simulink model "SystemIDsimulink"  (R2024b)
settings: Solver=ode5  StartTime=0.0  StopTime=20  FixedStep=.0005  RelTol=1e-3
undefined symbols (not defined in the file or in its folder): National_Instruments, PCIe
libraries: sldrtlib x4, slident x1, simulink x1
settings Model: Creator=jcglenn  LastModifiedBy=jcglenn
settings HardwareCC: ProdBitPerLong=64  ProdHWDeviceType=Intel->x86-64 (Linux 64)
settings RTWCC: Description=Simulink Desktop Real-Time  SystemTargetFile=sldrt.tlc  TemplateMakefile=sldrt.tmf  RTWCompilerOptimization=on
settings CodeAppCC: MaxIdLength=95
settings SimulinkDesktopRealTimeCC: TargetLibSuffix=_sldrt.a  TargetPreCompLibLocation=C:\Program Files\MATLAB\R2024b\toolbox\sldrt\lib\win64  ParMdlRefBuildCompliant=on

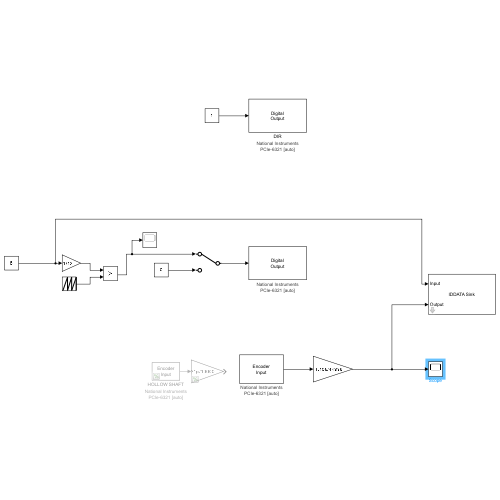
[thumbnail: Simulink's stored preview of the top-level diagram]
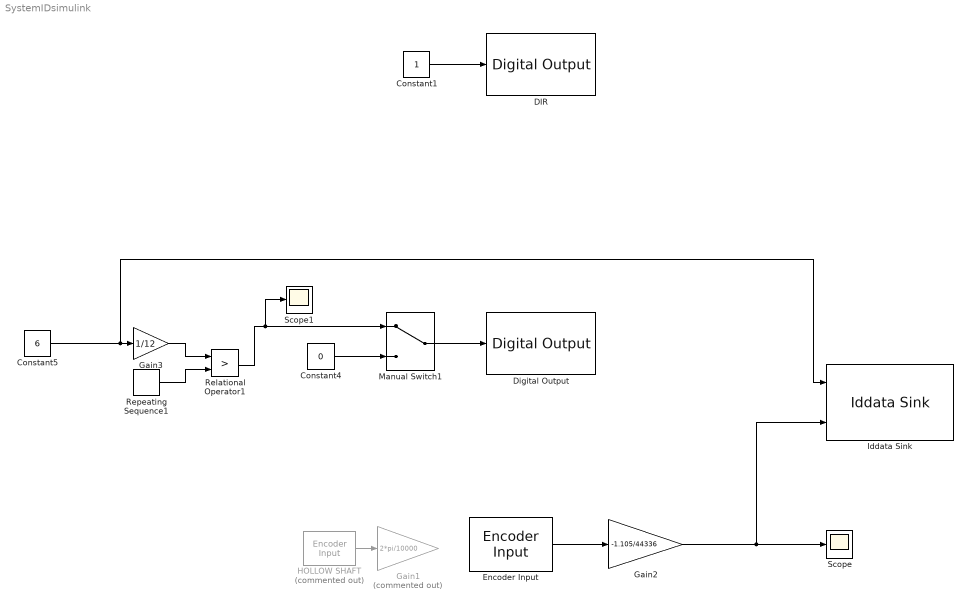
== system SystemIDsimulink ==
  Constant1 : Constant
  Constant4 : Constant  Value=0
  Constant5 : Constant  Value=6
  DIR : sldrtlib/Digital Output  SampleTime=0.0005  MaxMissedTicks=1000  ShowMissedTicks=off  YieldWhenWaiting=off  DrvName=National_Instruments/PCIe-6321  DrvAddress=4294967295  DrvOptions=[0 3 0 2 2 0 0]  Channels=2  BitMode=1  InitialValue=[]  FinalValue=[]
      settings: AttributesFormatString=National Instruments\nPCIe-6321 [auto]
  Digital Output : sldrtlib/Digital Output  SampleTime=0.0005  MaxMissedTicks=1000  ShowMissedTicks=off  YieldWhenWaiting=off  DrvName=National_Instruments/PCIe-6321  DrvAddress=4294967295  DrvOptions=[0 3 0 2 2 0 0]  Channels=1  BitMode=1  InitialValue=[]  FinalValue=[]
      settings: AttributesFormatString=National Instruments\nPCIe-6321 [auto]
  Encoder Input : sldrtlib/Encoder Input  SampleTime=0.0005  MaxMissedTicks=1000  ShowMissedTicks=off  YieldWhenWaiting=off  DrvName=National_Instruments/PCIe-6321  DrvAddress=4294967295  DrvOptions=[0 3 0 2 0 0 0]  Channels=1  QuadMode=3  IndexPulse=1  InputFilter=Inf  DataType=1
      settings: AttributesFormatString=National Instruments\nPCIe-6321 [auto]
  Gain1 : Gain  Commented=on  Gain=2*pi/10000
  Gain2 : Gain  Gain=-1.105/44336
  Gain3 : Gain  Gain=1/12
  HOLLOW SHAFT : sldrtlib/Encoder Input  Commented=on  SampleTime=0.01  MaxMissedTicks=10  ShowMissedTicks=off  YieldWhenWaiting=off  DrvName=National_Instruments/PCIe-6321  DrvAddress=4294967295  DrvOptions=[0 3 0 2 2 0 0]  Channels=2  QuadMode=3  IndexPulse=1  InputFilter=Inf  DataType=1
      settings: AttributesFormatString=National Instruments\nPCIe-6321 [auto]
  Iddata Sink : slident/Iddata Sink  datasetname=actuatorData  Ts=0.0005  isu=on  isy=on
  Manual Switch1 : ManualSwitch
  Relational Operator1 : RelationalOperator  Operator=>  OutDataTypeStr=boolean  RndMeth=Simplest  InputSameDT=off
  Repeating Sequence1 : simulink/Sources/Repeating Sequence  rep_seq_t=[0 .005]  rep_seq_y=[0 1]
  Scope : Scope
  Scope1 : Scope
  wires:
  Constant1/1 -> DIR/1
  Manual Switch1/1 -> Digital Output/1
  Encoder Input/1 -> Gain2/1
  Gain2/1 -> Scope/1, Iddata Sink/2
  Constant5/1 -> Iddata Sink/1, Gain3/1
  HOLLOW SHAFT/1 -> Gain1/1
  Repeating Sequence1/1 -> Relational Operator1/2
  Gain3/1 -> Relational Operator1/1
  Constant4/1 -> Manual Switch1/2
  Relational Operator1/1 -> Scope1/1, Manual Switch1/1
